simulink model "simulacoesCompensadores"  (R2020a)
settings: Solver=ode45  StartTime=0.0  StopTime=15  RelTol=1e-3  EnableMultiTasking=on
settings Model: Creator=20192610053  LastModifiedBy=batis
settings DataIOCC: LimitDataPoints=on  SaveFormat=Array  ReturnWorkspaceOutputs=off
settings OptimizationCC: LifeSpan=inf
settings DebuggingCC: SolverPrmCheckMsg=warning  SFUnexpectedBacktrackingDiag=warning  SFNoUnconditionalDefaultTransitionDiag=warning  SFExecutionAtInitializationDiag=none  ArithmeticOperatorsInVariantConditions=warning
settings HardwareCC: ProdBitPerPointer=32  ProdBitPerSizeT=32  ProdBitPerPtrDiffT=32  ProdLargestAtomicFloat=None  ProdIntDivRoundTo=Undefined  ProdEndianess=Unspecified  ProdWordSize=32  ProdHWDeviceType=32-bit Generic
settings ModelReferenceCC: PropagateSignalLabelsOutOfModel=off
settings SFSimCC: SimUseLocalCustomCode=off  CustomCodeUndefinedFunction=UseInterfaceOnly
settings RTWCC: RTWUseLocalCustomCode=off
settings CodeAppCC: StateflowObjectComments=on
settings GRTTargetCC: TargetLangStandard=C89/C90 (ANSI)
settings ConfigComp: CovMetricSettings=dw  CovHtmlReporting=on  CovSaveCumulativeToWorkspaceVar=on  CovSaveSingleToWorkspaceVar=on  CovExternalEMLEnable=off  CovSFcnEnable=off

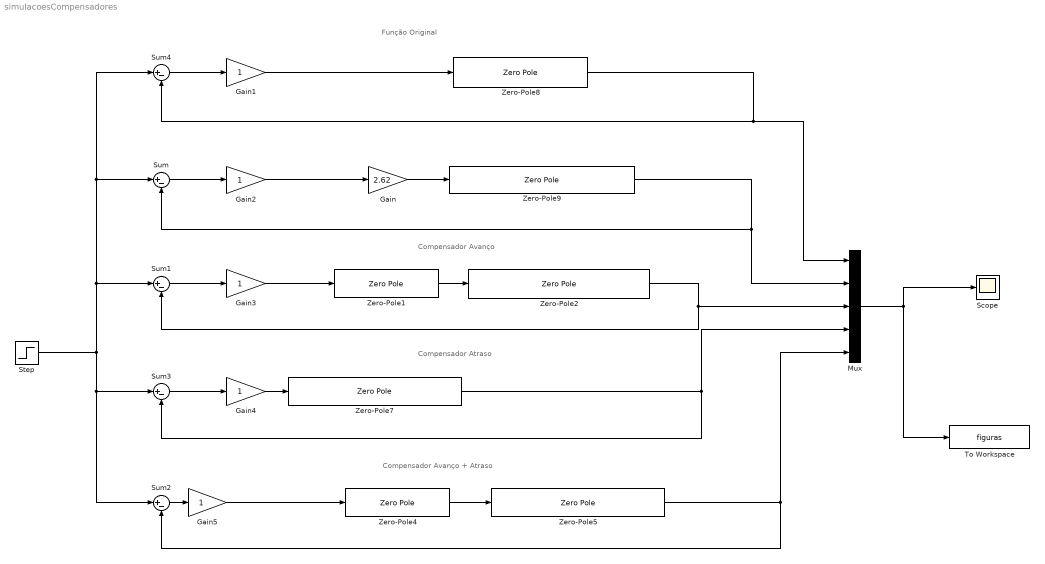
== system simulacoesCompensadores ==
  note: Compensador Avanço
  note: Função Original
  note: Compensador Atraso
  note: Compensador Avanço + Atraso
  Gain : Gain  Gain=2.62
  Gain{1..5} (5 alike) : Gain
  Mux : Mux  Inputs=5
  Scope : Scope
  Step : Step  Time=0  After=3  SampleTime=0
  Sum{,1..4} (5 alike) : Sum  Inputs=|+-
  To Workspace : ToWorkspace  VariableName=figuras  SampleTime=-1
      settings: Save2DSignal=2-D array (concatenate along first dimension)
  Zero-Pole1 : ZeroPole  Zeros=-0.8  Poles=[-0.77]  Gain=84.43
  Zero-Pole2 : ZeroPole  Zeros=[]  Poles=[-0.5 -11.05]  Gain=5.56
  Zero-Pole4 : ZeroPole  Zeros=-0.8  Poles=[-0.77]  Gain=84.43
  Zero-Pole5 : ZeroPole  Zeros=[-1.13]  Poles=[-0.00575 -0.5 -11.05]  Gain=14.51
  Zero-Pole7 : ZeroPole  Zeros=[-1.13]  Poles=[-0.00575 -0.5 -11.05]  Gain=14.51
  Zero-Pole8 : ZeroPole  Zeros=[]  Poles=[-0.5 -11.05]  Gain=5.56
  Zero-Pole9 : ZeroPole  Zeros=[]  Poles=[-0.5 -11.05]  Gain=5.56
  wires:
  Gain/1 -> Zero-Pole9/1
  Sum/1 -> Gain2/1
  Zero-Pole9/1 -> Mux/2, Sum/2
  Sum1/1 -> Gain3/1
  Zero-Pole1/1 -> Zero-Pole2/1
  Mux/1 -> To Workspace/1, Scope/1
  Sum2/1 -> Gain5/1
  Sum3/1 -> Gain4/1
  Zero-Pole2/1 -> Sum1/2, Mux/3
  Zero-Pole7/1 -> Mux/4, Sum3/2
  Zero-Pole5/1 -> Mux/5, Sum2/2
  Gain5/1 -> Zero-Pole4/1
  Gain1/1 -> Zero-Pole8/1
  Sum4/1 -> Gain1/1
  Zero-Pole8/1 -> Sum4/2, Mux/1
  Step/1 -> Sum1/1, Sum4/1, Sum/1, Sum2/1, Sum3/1
  Gain4/1 -> Zero-Pole7/1
  Gain3/1 -> Zero-Pole1/1
  Gain2/1 -> Gain/1
  Zero-Pole4/1 -> Zero-Pole5/1
